simulink model "dspdtmf_audio"  (Simulink 8.3)
settings: Solver=FixedStepDiscrete  SolverMode=SingleTasking  StartTime=0  StopTime=5  RelTol=1e-3
model workspace (MAT data in the model file):
  dtmfFramesize = 256
  dtmfFs : num (value not decoded)
undefined symbols (not defined in the file or in its folder): dfilt, jet
libraries: dspsrcs4 x7, dspsigops x2, dspsnks4 x2, dspobslib x1, dsparch4 x1, dspswit3 x1, dspbuff3 x1, dspmisc x1, dspspect3 x1, dspmathops x1
settings Model: FPTRunName=Active  Creator=The MathWorks Inc.  ExtModeTrigMode=oneshot  ExtModeArmWhenConnect=off  ExtModeAutoUpdateStatusClock=off  BufferReuse=off
settings DataIOCC: LimitDataPoints=off  SaveOutput=off  SignalLogging=off  SaveTime=off
settings OptimizationCC: BlockReduction=off  BooleanDataType=off  OptimizeBlockIOStorage=off  BufferReuse=off  GlobalBufferReuse=off  ExpressionFolding=off  ExpressionDepthLimit=2147483647  FoldNonRolledExpr=off  LocalBlockOutputs=off  InitFltsAndDblsToZero=on
settings DebuggingCC: SignalResolutionControl=TryResolveAllWithWarning  SolverPrmCheckMsg=none  MultiTaskDSMMsg=warning  MultiTaskCondExecSysMsg=none  FcnCallInpInsideContextMsg=UseLocalSettings  StrictBusMsg=None
settings HardwareCC: TargetUnknown=on
settings SFSimCC: SimParseCustomCode=off
settings RTWCC: IncludeERTFirstTime=on
settings GRTTargetCC: TargetFcnLib=ansi_tfl_tmw_new.mat

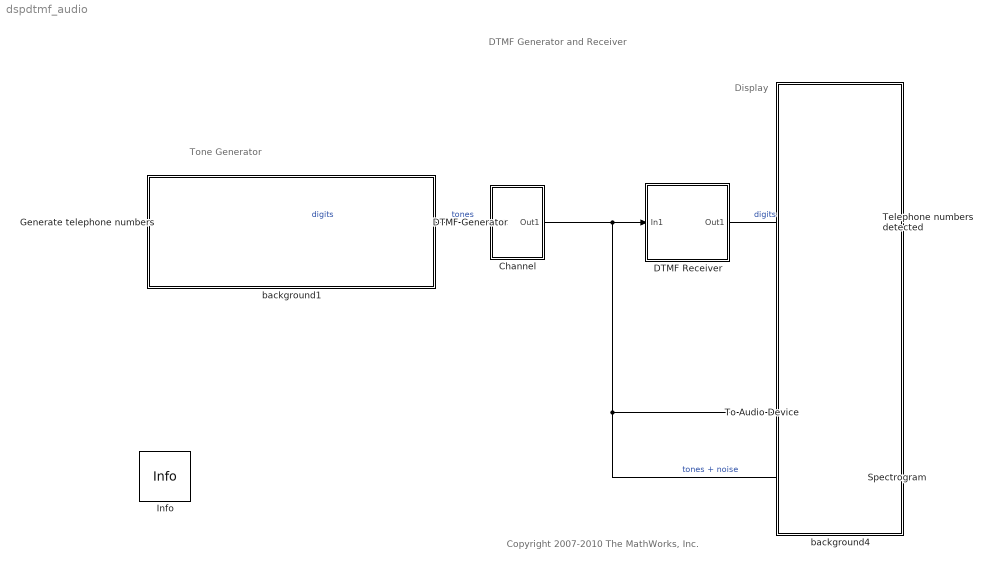
== system dspdtmf_audio ==
  note: DTMF Generator and Receiver
  note: Display
  note: Tone
      | Generator
  note: Copyright 2007-2010 The MathWorks, Inc.
  Channel : Subsystem  mask(Channel){var=0.04, g=2}
      mask prompts: var "Noise power"; g "Gain"
      mask help: Models a noisy channel
      mask Display: disp('Channel')
  DTMF Generator : Subsystem  mask(DTMF Generator){dtmfdelta_f1=4.5, dtmfdelta_f2=0, dtmfdelta_f3=0, dtmfdelta_f4=0, dtmfdelta_f5=0, dtmfdelta_f6=0, dtmfdelta_f7=0}
      mask prompts: dtmfdelta_f1 "Row tone 1 (697 Hz) frequency bias (%):"; dtmfdelta_f2 "Row tone 2 (770 Hz) frequency bias (%):"; dtmfdelta_f3 "Row tone 3 (852 Hz) frequency bias (%):"; dtmfdelta_f4 "Row tone 4 (941 Hz) frequency bias (%):"; dtmfdelta_f5 "Column tone 1 (1209 Hz) frequency bias (%):"; dtmfdelta_f6 "Column tone 2 (1336 Hz) frequency bias (%):"; dtmfdelta_f7 "Column tone 3 (1477 Hz) frequency bias (%):"
      mask help: Generates dual-tone multifrequency tones by summing row and column frequency tones. The frequency bias of each row and column frequency tone can be specified as a percentage of the tone frequency.
      mask Display: disp('DTMF\nGenerator');
  DTMF Receiver : Subsystem  mask(DTMF Receiver){dtmf_p=4.5}
      mask prompts: dtmf_p "Bandpass filter frequency bandwidth (% of central frequency):"
      mask help: Receiver and decoder for dual-tone multifrequency tones. The bandwidth of the bandpass filters can be specified as a percentage of the center frequency.
      mask Display: disp('DTMF\nReceiver');
  Generate telephone numbers : Subsystem  mask{Number=[1 5 0 8 6 4 7 7 0 0 0], Td=(1/dtmfFs)*256*6}
      mask prompts: Number "Telephone number"; Td "Digit Period (s)"
      mask help: This block simulates the dialed numbers. The output is a sequency of pulses with the dialed number as the pulse amplitude.
      mask init:
      | if (~isreal(Number) || ~isvector(Number) || issparse(Number) || ischar(Number) || isfi(Number))
      |     error(['Input must be an integer vector with values in the range 0 to 11, inclusive']);
      | end
      | for i = 1:length(Number)
      |     if ((Number(i) > 11) || (Number(i)<0)) || ((Number(i)-floor(Number(i)))~=0)
      |         error(['Input values must be integers from 0 to 11, inclusive']);
      |     end
      | end
      mask Display: disp(Number)
  Info : dspmisc/Info  SystemSampleTime=-1
  Spectrogram : Subsystem
  Telephone numbers detected : Display
  To Audio Device : dspsnks4/To Audio Device  deviceName=Default  inheritSampleRate=on  sampleRate=44100  deviceDatatype=Determine from input data type  autoBufferSize=on  bufferSize=4096  queueDuration=0.3  defaultOutputChannelMapping=on  outputChannelMapping=1
  background1 : Subsystem
      mask Display: disp('')
  background4 : Subsystem
      mask Display: disp('')
  wires:
  Generate telephone numbers/1(Out1) -> DTMF Generator/1(In1)  "digits"
  Channel/1(Out1) -> DTMF Receiver/1(In1), Spectrogram/1(In1), To Audio Device/1  "tones + noise"
  DTMF Receiver/1(Out1) -> Telephone numbers detected/1  "digits"
  DTMF Generator/1(Out1) -> Channel/1(In1)  "tones"

== system dspdtmf_audio/Channel ==
  In1 : Inport
  Gain : Gain  Gain=g  SaturateOnIntegerOverflow=on  OutDataTypeStr=Inherit: Same as input  ParamDataTypeStr=Inherit: Same as input
  Sum : Sum  Inputs=|++  SaturateOnIntegerOverflow=on  InputSameDT=on  OutDataTypeStr=Inherit: Same as first input
  Vector of Noise : RandomNumber  Variance=var  Seed=[1:dtmfFramesize]  SampleTime=dtmfFramesize/dtmfFs
  Out1 : Outport
  wires:
  In1/1 -> Gain/1
  Gain/1 -> Sum/1
  Vector of Noise/1 -> Sum/2
  Sum/1 -> Out1/1

== system dspdtmf_audio/DTMF Generator ==
  In1 : Inport
  Constant : Constant
  Digit to Tone : Subsystem  TreatAsAtomicUnit=on
  Sum : Sum  Inputs=|+-  SaturateOnIntegerOverflow=on  InputSameDT=on  OutDataTypeStr=Inherit: Same as first input
  Out1 : Outport
  wires:
  In1/1 -> Digit to Tone/Enable, Sum/1
  Sum/1 -> Digit to Tone/1(In1)
  Constant/1 -> Sum/2
  Digit to Tone/1(Out1) -> Out1/1

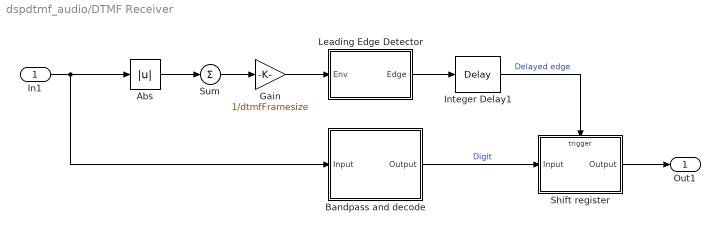
== system dspdtmf_audio/DTMF Receiver ==
  In1 : Inport
  Abs : Abs  SaturateOnIntegerOverflow=on
  Bandpass and decode : Subsystem
  Gain : Gain  Gain=1/dtmfFramesize  SaturateOnIntegerOverflow=on  OutDataTypeStr=Inherit: Same as input  ParamDataTypeStr=Inherit: Same as input
  Integer Delay1 : dspsigops/Delay  dly_unit=Samples  delay=1  ic_detail=off  dif_ic_for_ch=off  dif_ic_for_dly=off  ic=0  reset_popup=None
  Leading Edge Detector : Subsystem
  Shift register : Subsystem  TreatAsAtomicUnit=on
  Sum : Sum  Inputs=1  SaturateOnIntegerOverflow=on  InputSameDT=on  OutDataTypeStr=Inherit: Same as first input
  Out1 : Outport
  wires:
  In1/1 -> Bandpass and decode/1(Input), Abs/1
  Abs/1 -> Sum/1
  Sum/1 -> Gain/1
  Gain/1 -> Leading Edge Detector/1(Env)
  Leading Edge Detector/1(Edge) -> Integer Delay1/1
  Bandpass and decode/1(Output) -> Shift register/1(Input)  "Digit"
  Integer Delay1/1 -> Shift register/Trigger  "Delayed edge"
  Shift register/1(Output) -> Out1/1

== system dspdtmf_audio/Generate telephone numbers ==
  Discrete Pulse Generator : DiscretePulseGenerator  SampleTime=Td
  Product : Product  SaturateOnIntegerOverflow=on  RndMeth=Zero  InputSameDT=on  OutDataTypeStr=Inherit: Same as first input
  Triggered Signal From Workspace1 : dspsigops/Triggered Signal From Workspace  Signal=Number+1  TriggerType=Rising edge  ic=0  SamplesPerFrame=1  OutputAfterFinalValue=Setting to zero
  Out1 : Outport
  wires:
  Discrete Pulse Generator/1 -> Product/1, Triggered Signal From Workspace1/Trigger
  Triggered Signal From Workspace1/1 -> Product/2
  Product/1 -> Out1/1

== system dspdtmf_audio/Spectrogram ==
  In1 : Inport
  Buffer2 : Buffer  N=48*64  V=46*64  ic=-70  TreatMby1Signals=One channel
  Reshape : Reshape  OutputDimensionality=Customize  OutputDimensions=[64 48]
  Selector : Selector  InputPortWidth=dtmfFramesize/2  Indices=1:(dtmfFramesize/4)
  Short-Time FFT1 : dspspect3/Periodogram  measurement=Power spectral density  wintype=Hamming  Rs=50  beta=5  winsamp=Periodic  FFTImplementation=Auto  inheritFFT=off  fftsize=128  navg=2  inheritTs=on  Ts=1
  Spectogram : dspsnks4/Matrix Viewer  ImageParams=on  CMapStr=jet(256)  AxisColorbar=off  AxisParams=on  AxisOrigin=Lower left corner  XLabel=Time Index  YLabel=Frequency Index  ZLabel=dB Magnitude  FigPos=[214 452 283 114]  AxisZoom=on
      settings: YMin=-150  YMax=-65
  dB Conversion : dspmathops/dB Conversion  dBtype=dB  intype=Amplitude  R=1  fuzz=on
  wires:
  Short-Time FFT1/1 -> Selector/1
  Selector/1 -> dB Conversion/1
  Buffer2/1 -> Reshape/1
  In1/1 -> Short-Time FFT1/1
  Reshape/1 -> Spectogram/1
  dB Conversion/1 -> Buffer2/1

== system dspdtmf_audio/background1 ==

== system dspdtmf_audio/background4 ==

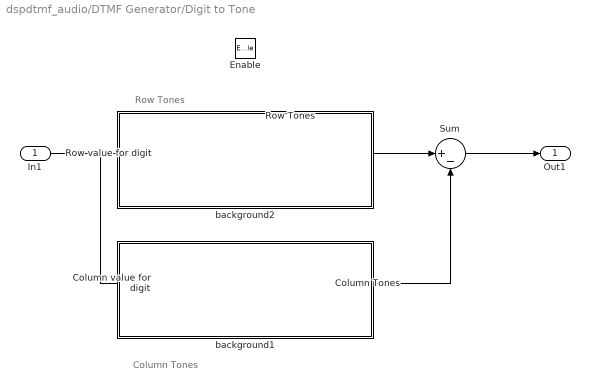
== system dspdtmf_audio/DTMF Generator/Digit to Tone ==
  note: Row Tones
  note: Column Tones
  In1 : Inport
  Enable : EnablePort  PropagateVarSize=During execution
  Column Tones : Subsystem
  Column value for digit : Lookup_n-D  NumberOfTableDimensions=1  BreakpointsForDimension1=[0 1 2 3 4 5 6 7 8 9 10 11]  Table=[1 0 1 2 0 1 2 0 1 2 0 2]  SaturateOnIntegerOverflow=on  InputSameDT=on
  Row Tones : Subsystem
  Row value for digit : Lookup_n-D  NumberOfTableDimensions=1  BreakpointsForDimension1=[0 1 2 3 4 5 6 7 8 9 10 11]  Table=[3 0 0 0 1 1 1 2 2 2 3 3]  SaturateOnIntegerOverflow=on  InputSameDT=on
  Sum : Sum  Inputs=|+-  SaturateOnIntegerOverflow=on  InputSameDT=on  OutDataTypeStr=Inherit: Same as first input
  background1 : Subsystem
      mask Display: disp('')
  background2 : Subsystem
      mask Display: disp('')
  Out1 : Outport  OutputWhenDisabled=reset  InitialOutput=0
  wires:
  Sum/1 -> Out1/1
  Column value for digit/1 -> Column Tones/1(Column)
  Row value for digit/1 -> Row Tones/1(Row)
  In1/1 -> Column value for digit/1, Row value for digit/1
  Column Tones/1(Tone) -> Sum/2
  Row Tones/1(Tone) -> Sum/1

== system dspdtmf_audio/DTMF Receiver/Bandpass and decode ==
  Input : Inport
  Calculate Digit : Lookup_n-D  BreakpointsForDimension1=[1:4]  BreakpointsForDimension2=[1:3]  Table=[1 2 3;4 5 6;7 8 9;10 0 11]  ExtrapMethod=Clip  SaturateOnIntegerOverflow=on  InputSameDT=on
  Calculate Column : Subsystem
  Calculate Row : Subsystem
  Output : Outport
  wires:
  Input/1 -> Calculate Column/1(In1), Calculate Row/1(In1)  "Input Tones"
  Calculate Digit/1 -> Output/1
  Calculate Row/1(Out1) -> Calculate Digit/1
  Calculate Column/1(Out1) -> Calculate Digit/2

== system dspdtmf_audio/DTMF Receiver/Leading Edge Detector ==
  Env : Inport
  Binary To Bipolar : Fcn  Expr=2*u-1
  Constant : Constant  Value=0.5
  Digital Filter : dsparch4/Digital Filter  TypePopup=FIR (all zeros)  IIRFiltStruct=Direct form II transposed  AllPoleFiltStruct=Direct form  FIRFiltStruct=Direct form  CoeffSource=Specify via dialog  NumCoeffs=[ones(1,4) -ones(1,4)]  DenCoeffs=[1 0.1]  BiQuadCoeffs=[1 0.3 0.4 1 0.1 0.2]  LatticeCoeffs=[0.2 0.4]  denIgnore=on  FiltPerSampPopup=One filter per frame  IC=0  ICnum=0  ICden=0  roundingMode=Floor  overflowMode=off  ScaleValues=1  scaleValueFracLength=14  stageInFracLength=15  stageOutFracLength=15  FilterSource=Specify via dialog  dfiltObjectName=dfilt.dffir([1 2 1])
  Edge Detector1 : dspswit3/Edge Detector
  Relational Operator : RelationalOperator  InputSameDT=on
  Rising Edge Start : Fcn  Expr=u>5
  Edge : Outport
  wires:
  Edge Detector1/1 -> Edge/1
  Digital Filter/1 -> Rising Edge Start/1
  Binary To Bipolar/1 -> Digital Filter/1
  Rising Edge Start/1 -> Edge Detector1/1
  Env/1 -> Relational Operator/1
  Constant/1 -> Relational Operator/2
  Relational Operator/1 -> Binary To Bipolar/1

== system dspdtmf_audio/DTMF Receiver/Shift register ==
  Input : Inport
  Trigger : TriggerPort  ZeroCross=off
  Delay Line : dspbuff3/Delay Line  siz=11  ic=0  directfeed=on  enable_output=off  hold_output=off  TreatMby1Signals=One channel
  Output : Outport
  wires:
  Input/1 -> Delay Line/1
  Delay Line/1 -> Output/1

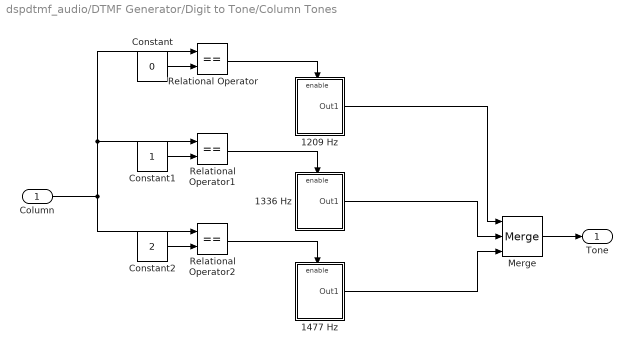
== system dspdtmf_audio/DTMF Generator/Digit to Tone/Column Tones ==
  Column : Inport
  1209 Hz : Subsystem  TreatAsAtomicUnit=on
  1336 Hz : Subsystem  TreatAsAtomicUnit=on
  1477 Hz : Subsystem  TreatAsAtomicUnit=on
  Constant : Constant  Value=0
  Constant1 : Constant
  Constant2 : Constant  Value=2
  Merge : Merge  Inputs=3
  Relational Operator : RelationalOperator  Operator===  InputSameDT=on
  Relational Operator1 : RelationalOperator  Operator===  InputSameDT=on
  Relational Operator2 : RelationalOperator  Operator===  InputSameDT=on
  Tone : Outport
  wires:
  Merge/1 -> Tone/1
  1477 Hz/1(Out1) -> Merge/3
  1336 Hz/1(Out1) -> Merge/2
  1209 Hz/1(Out1) -> Merge/1
  Column/1 -> Relational Operator/1, Relational Operator1/1, Relational Operator2/1
  Relational Operator/1 -> 1209 Hz/Enable
  Relational Operator1/1 -> 1336 Hz/Enable
  Relational Operator2/1 -> 1477 Hz/Enable
  Constant/1 -> Relational Operator/2
  Constant1/1 -> Relational Operator1/2
  Constant2/1 -> Relational Operator2/2

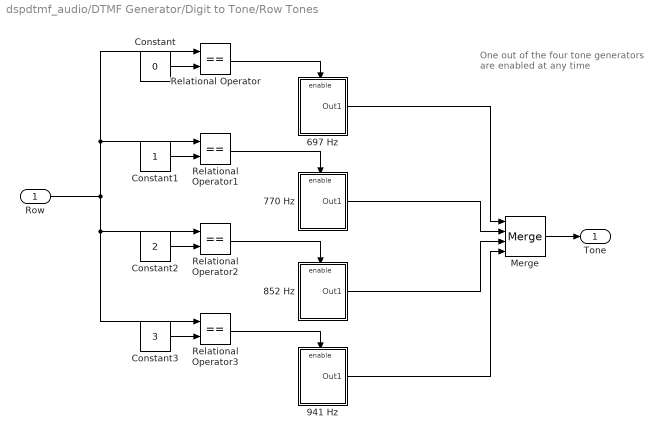
== system dspdtmf_audio/DTMF Generator/Digit to Tone/Row Tones ==
  note: One out of the four tone generators
      | are enabled at any time
  Row : Inport
  697 Hz : Subsystem  TreatAsAtomicUnit=on
  770 Hz : Subsystem  TreatAsAtomicUnit=on
  852 Hz : Subsystem  TreatAsAtomicUnit=on
  941 Hz : Subsystem  TreatAsAtomicUnit=on
  Constant : Constant  Value=0
  Constant1 : Constant
  Constant2 : Constant  Value=2
  Constant3 : Constant  Value=3
  Merge : Merge  Inputs=4
  Relational Operator{,1..3} (4 alike) : RelationalOperator  Operator===  InputSameDT=on
  Tone : Outport
  wires:
  Row/1 -> Relational Operator/1, Relational Operator1/1, Relational Operator2/1, Relational Operator3/1
  697 Hz/1(Out1) -> Merge/1
  770 Hz/1(Out1) -> Merge/2
  852 Hz/1(Out1) -> Merge/3
  941 Hz/1(Out1) -> Merge/4
  Merge/1 -> Tone/1
  Relational Operator/1 -> 697 Hz/Enable
  Relational Operator1/1 -> 770 Hz/Enable
  Relational Operator2/1 -> 852 Hz/Enable
  Relational Operator3/1 -> 941 Hz/Enable
  Constant/1 -> Relational Operator/2
  Constant1/1 -> Relational Operator1/2
  Constant2/1 -> Relational Operator2/2
  Constant3/1 -> Relational Operator3/2

== system dspdtmf_audio/DTMF Generator/Digit to Tone/background1 ==

== system dspdtmf_audio/DTMF Generator/Digit to Tone/background2 ==

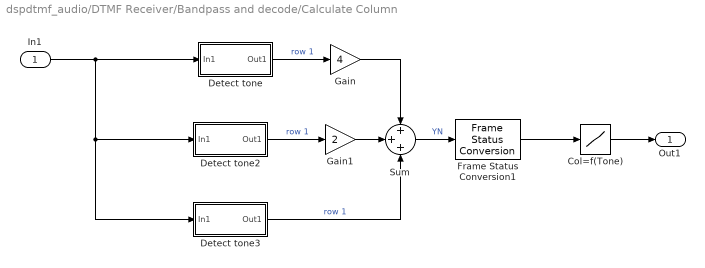
== system dspdtmf_audio/DTMF Receiver/Bandpass and decode/Calculate Column ==
  In1 : Inport
  Col=f(Tone) : Lookup_n-D  NumberOfTableDimensions=1  BreakpointsForDimension1=[0:7]  Table=[0 1 2 0 3 0 0 0]  SaturateOnIntegerOverflow=on  InputSameDT=on
  Detect tone : Subsystem  mask{F=1477}
      mask prompts: F "Frequency"
      settings: AttributesFormatString=%<F> Hz
  Detect tone2 : Subsystem  mask{F=1336}
      mask prompts: F "Frequency"
      settings: AttributesFormatString=%<F> Hz
  Detect tone3 : Subsystem  mask{F=1209}
      mask prompts: F "Frequency"
      settings: AttributesFormatString=%<F> Hz
  Frame Status Conversion1 : dspobslib/Frame Status Conversion  growRefPort=off  outframe=Sample-based
  Gain : Gain  Gain=4
  Gain1 : Gain  Gain=2
  Sum : Sum  Inputs=+++
  Out1 : Outport
  wires:
  Sum/1 -> Frame Status Conversion1/1  "YN"
  Frame Status Conversion1/1 -> Col=f(Tone)/1
  Detect tone2/1(Out1) -> Gain1/1  "row 1"
  In1/1 -> Detect tone/1(In1), Detect tone3/1(In1), Detect tone2/1(In1)
  Col=f(Tone)/1 -> Out1/1
  Gain1/1 -> Sum/2
  Detect tone/1(Out1) -> Gain/1  "row 1"
  Gain/1 -> Sum/1
  Detect tone3/1(Out1) -> Sum/3  "row 1"

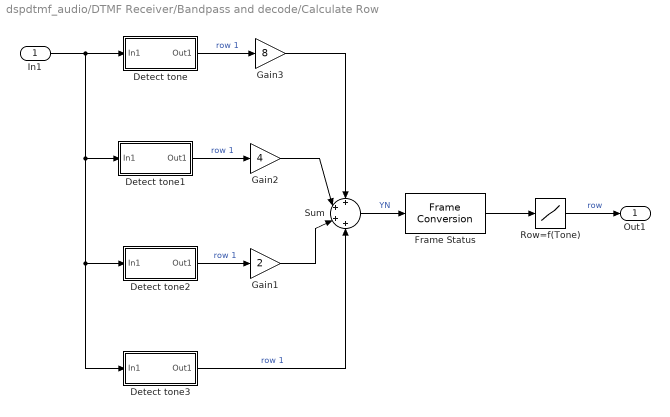
== system dspdtmf_audio/DTMF Receiver/Bandpass and decode/Calculate Row ==
  In1 : Inport
  Detect tone : Subsystem  mask{F=941}
      mask prompts: F "Frequency"
      settings: AttributesFormatString=%<F> Hz
  Detect tone1 : Subsystem  mask{F=852}
      mask prompts: F "Frequency"
      settings: AttributesFormatString=%<F> Hz
  Detect tone2 : Subsystem  mask{F=770}
      mask prompts: F "Frequency"
      settings: AttributesFormatString=%<F> Hz
  Detect tone3 : Subsystem  mask{F=697}
      mask prompts: F "Frequency"
      settings: AttributesFormatString=%<F> Hz
  Frame Status : FrameConversion  OutFrame=Sample-based
  Gain1 : Gain  Gain=2
  Gain2 : Gain  Gain=4
  Gain3 : Gain  Gain=8
  Row=f(Tone) : Lookup_n-D  NumberOfTableDimensions=1  BreakpointsForDimension1=[0:15]  Table=[0 1 2 0 3 0 0 0 4 0 0 0 0 0 0 0]  SaturateOnIntegerOverflow=on  InputSameDT=on
  Sum : Sum  Inputs=++++
  Out1 : Outport
  wires:
  In1/1 -> Detect tone/1(In1), Detect tone1/1(In1), Detect tone2/1(In1), Detect tone3/1(In1)
  Row=f(Tone)/1 -> Out1/1  "row"
  Frame Status/1 -> Row=f(Tone)/1
  Detect tone2/1(Out1) -> Gain1/1  "row 1"
  Detect tone1/1(Out1) -> Gain2/1  "row 1"
  Detect tone/1(Out1) -> Gain3/1  "row 1"
  Gain3/1 -> Sum/1
  Gain2/1 -> Sum/2
  Gain1/1 -> Sum/3
  Sum/1 -> Frame Status/1  "YN"
  Detect tone3/1(Out1) -> Sum/4  "row 1"

== system dspdtmf_audio/DTMF Generator/Digit to Tone/Column Tones/1209 Hz ==
  Enable : EnablePort  PropagateVarSize=During execution
  Sine Wave1 : dspsrcs4/Sine Wave  Amplitude=1  Frequency=1209*(1+dtmfdelta_f5/100)  Phase=0  SampleMode=Discrete  OutComplex=Real  CompMethod=Trigonometric fcn  TableSize=Speed  SampleTime=1/dtmfFs  SamplesPerFrame=dtmfFramesize  ResetState=Restart at time zero  dataType=double  wordLen=16  udDataType=sfix(16)  fracBitsMode=Best precision  numFracBits=15  OutDataTypeStr=double  LastOutDataTypeStr=double
  Out1 : Outport
  wires:
  Sine Wave1/1 -> Out1/1

== system dspdtmf_audio/DTMF Generator/Digit to Tone/Column Tones/1336 Hz ==
  Enable : EnablePort  PropagateVarSize=During execution
  Sine Wave1 : dspsrcs4/Sine Wave  Amplitude=1  Frequency=1336*(1+dtmfdelta_f6/100)  Phase=0  SampleMode=Discrete  OutComplex=Real  CompMethod=Trigonometric fcn  TableSize=Speed  SampleTime=1/dtmfFs  SamplesPerFrame=dtmfFramesize  ResetState=Restart at time zero  dataType=double  wordLen=16  udDataType=sfix(16)  fracBitsMode=Best precision  numFracBits=15  OutDataTypeStr=double  LastOutDataTypeStr=double
  Out1 : Outport
  wires:
  Sine Wave1/1 -> Out1/1

== system dspdtmf_audio/DTMF Generator/Digit to Tone/Column Tones/1477 Hz ==
  Enable : EnablePort  PropagateVarSize=During execution
  Sine Wave1 : dspsrcs4/Sine Wave  Amplitude=1  Frequency=1477*(1+dtmfdelta_f7/100)  Phase=0  SampleMode=Discrete  OutComplex=Real  CompMethod=Trigonometric fcn  TableSize=Speed  SampleTime=1/dtmfFs  SamplesPerFrame=dtmfFramesize  ResetState=Restart at time zero  dataType=double  wordLen=16  udDataType=sfix(16)  fracBitsMode=Best precision  numFracBits=15  OutDataTypeStr=double  LastOutDataTypeStr=double
  Out1 : Outport
  wires:
  Sine Wave1/1 -> Out1/1

== system dspdtmf_audio/DTMF Generator/Digit to Tone/Row Tones/697 Hz ==
  Enable : EnablePort  PropagateVarSize=During execution
  Sine Wave : dspsrcs4/Sine Wave  Amplitude=1  Frequency=697*(1+dtmfdelta_f1/100)  Phase=0  SampleMode=Discrete  OutComplex=Real  CompMethod=Trigonometric fcn  TableSize=Speed  SampleTime=1/dtmfFs  SamplesPerFrame=dtmfFramesize  ResetState=Restart at time zero  dataType=double  wordLen=16  udDataType=sfix(16)  fracBitsMode=Best precision  numFracBits=15  OutDataTypeStr=double  LastOutDataTypeStr=double
  Out1 : Outport
  wires:
  Sine Wave/1 -> Out1/1

== system dspdtmf_audio/DTMF Generator/Digit to Tone/Row Tones/770 Hz ==
  Enable : EnablePort  PropagateVarSize=During execution
  Sine Wave : dspsrcs4/Sine Wave  Amplitude=1  Frequency=770*(1+dtmfdelta_f2/100)  Phase=0  SampleMode=Discrete  OutComplex=Real  CompMethod=Trigonometric fcn  TableSize=Speed  SampleTime=1/dtmfFs  SamplesPerFrame=dtmfFramesize  ResetState=Restart at time zero  dataType=double  wordLen=16  udDataType=sfix(16)  fracBitsMode=Best precision  numFracBits=15  OutDataTypeStr=double  LastOutDataTypeStr=double
  Out1 : Outport
  wires:
  Sine Wave/1 -> Out1/1

== system dspdtmf_audio/DTMF Generator/Digit to Tone/Row Tones/852 Hz ==
  Enable : EnablePort  PropagateVarSize=During execution
  Sine Wave : dspsrcs4/Sine Wave  Amplitude=1  Frequency=852*(1+dtmfdelta_f3/100)  Phase=0  SampleMode=Discrete  OutComplex=Real  CompMethod=Trigonometric fcn  TableSize=Speed  SampleTime=1/dtmfFs  SamplesPerFrame=dtmfFramesize  ResetState=Restart at time zero  dataType=double  wordLen=16  udDataType=sfix(16)  fracBitsMode=Best precision  numFracBits=15  OutDataTypeStr=double  LastOutDataTypeStr=double
  Out1 : Outport
  wires:
  Sine Wave/1 -> Out1/1

== system dspdtmf_audio/DTMF Generator/Digit to Tone/Row Tones/941 Hz ==
  Enable : EnablePort  PropagateVarSize=During execution
  Sine Wave : dspsrcs4/Sine Wave  Amplitude=1  Frequency=941*(1+dtmfdelta_f4/100)  Phase=0  SampleMode=Discrete  OutComplex=Real  CompMethod=Trigonometric fcn  TableSize=Speed  SampleTime=1/dtmfFs  SamplesPerFrame=dtmfFramesize  ResetState=Restart at time zero  dataType=double  wordLen=16  udDataType=sfix(16)  fracBitsMode=Best precision  numFracBits=15  OutDataTypeStr=double  LastOutDataTypeStr=double
  Out1 : Outport
  wires:
  Sine Wave/1 -> Out1/1

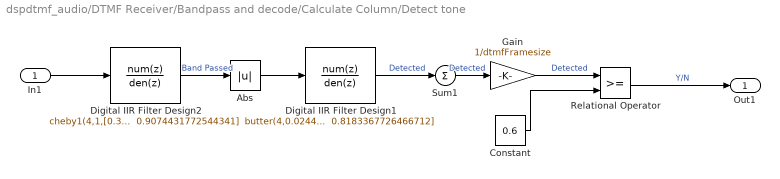
== system dspdtmf_audio/DTMF Receiver/Bandpass and decode/Calculate Column/Detect tone ==
  In1 : Inport
  Abs : Abs  SaturateOnIntegerOverflow=on
  Constant : Constant  Value=0.6
  Digital IIR Filter Design1 : DiscreteFilter  Numerator=butter(4,0.024414 )  Denominator="[1     -3.799600047139706      5.418636382695164      -3.43734174118743     0.8183367726466712]"  InputProcessing=Columns as channels (frame based)
  Digital IIR Filter Design2 : DiscreteFilter  Numerator=cheby1(4,1,[0.34437 0.37682] )  Denominator="[1     -3.351534504625169       8.10699128745984     -12.15068111449483      14.40624674632962     -11.85923479241394      7.722756593485457     -3.116033501354059     0.9074431772544341]"  InputProcessing=Columns as channels (frame based)
  Gain : Gain  Gain=1/dtmfFramesize  SaturateOnIntegerOverflow=on  OutDataTypeStr=Inherit: Same as input  ParamDataTypeStr=Inherit: Same as input
  Relational Operator : RelationalOperator  InputSameDT=on
  Sum1 : Sum  Inputs=1  SaturateOnIntegerOverflow=on  InputSameDT=on  OutDataTypeStr=Inherit: Same as first input
  Out1 : Outport
  wires:
  Digital IIR Filter Design1/1 -> Sum1/1  "Detected"
  Relational Operator/1 -> Out1/1  "Y/N"
  Constant/1 -> Relational Operator/2
  Abs/1 -> Digital IIR Filter Design1/1
  Digital IIR Filter Design2/1 -> Abs/1  "Band Passed"
  In1/1 -> Digital IIR Filter Design2/1
  Sum1/1 -> Gain/1  "Detected"
  Gain/1 -> Relational Operator/1  "Detected"

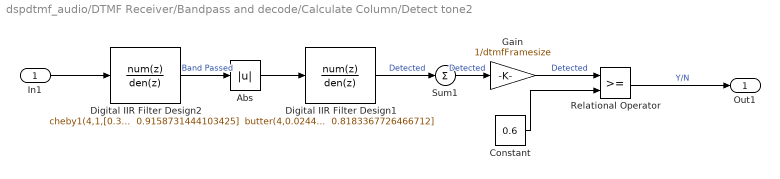
== system dspdtmf_audio/DTMF Receiver/Bandpass and decode/Calculate Column/Detect tone2 ==
  In1 : Inport
  Abs : Abs  SaturateOnIntegerOverflow=on
  Constant : Constant  Value=0.6
  Digital IIR Filter Design1 : DiscreteFilter  Numerator=butter(4,0.024414 )  Denominator="[1     -3.799600047139706      5.418636382695164      -3.43734174118743     0.8183367726466712]"  InputProcessing=Columns as channels (frame based)
  Digital IIR Filter Design2 : DiscreteFilter  Numerator=cheby1(4,1,[0.31149 0.34085] )  Denominator="[1     -4.109271737397858      10.23854068371831     -16.38274148509198      19.22475767149518     -16.02675157800493      9.798412568107882     -3.847129397590863     0.9158731444103425]"  InputProcessing=Columns as channels (frame based)
  Gain : Gain  Gain=1/dtmfFramesize  SaturateOnIntegerOverflow=on  OutDataTypeStr=Inherit: Same as input  ParamDataTypeStr=Inherit: Same as input
  Relational Operator : RelationalOperator  InputSameDT=on
  Sum1 : Sum  Inputs=1  SaturateOnIntegerOverflow=on  InputSameDT=on  OutDataTypeStr=Inherit: Same as first input
  Out1 : Outport
  wires:
  Gain/1 -> Relational Operator/1  "Detected"
  Sum1/1 -> Gain/1  "Detected"
  In1/1 -> Digital IIR Filter Design2/1
  Digital IIR Filter Design2/1 -> Abs/1  "Band Passed"
  Abs/1 -> Digital IIR Filter Design1/1
  Constant/1 -> Relational Operator/2
  Relational Operator/1 -> Out1/1  "Y/N"
  Digital IIR Filter Design1/1 -> Sum1/1  "Detected"

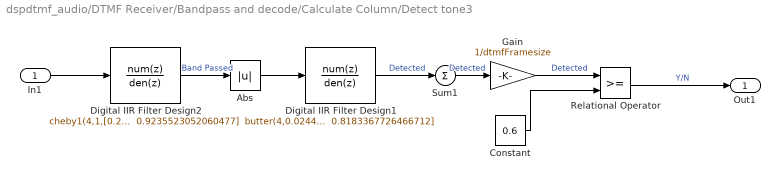
== system dspdtmf_audio/DTMF Receiver/Bandpass and decode/Calculate Column/Detect tone3 ==
  In1 : Inport
  Abs : Abs  SaturateOnIntegerOverflow=on
  Constant : Constant  Value=0.6
  Digital IIR Filter Design1 : DiscreteFilter  Numerator=butter(4,0.024414 )  Denominator="[1     -3.799600047139706      5.418636382695164      -3.43734174118743     0.8183367726466712]"  InputProcessing=Columns as channels (frame based)
  Digital IIR Filter Design2 : DiscreteFilter  Numerator=cheby1(4,1,[0.28188 0.30845] )  Denominator="[1     -4.752348043106542      12.38564406749955     -20.67287188883259      24.34715829142214     -20.26589425714094      11.90277663892072     -4.477143154545357     0.9235523052060477]"  InputProcessing=Columns as channels (frame based)
  Gain : Gain  Gain=1/dtmfFramesize  SaturateOnIntegerOverflow=on  OutDataTypeStr=Inherit: Same as input  ParamDataTypeStr=Inherit: Same as input
  Relational Operator : RelationalOperator  InputSameDT=on
  Sum1 : Sum  Inputs=1  SaturateOnIntegerOverflow=on  InputSameDT=on  OutDataTypeStr=Inherit: Same as first input
  Out1 : Outport
  wires:
  Digital IIR Filter Design1/1 -> Sum1/1  "Detected"
  Relational Operator/1 -> Out1/1  "Y/N"
  Constant/1 -> Relational Operator/2
  Abs/1 -> Digital IIR Filter Design1/1
  Digital IIR Filter Design2/1 -> Abs/1  "Band Passed"
  In1/1 -> Digital IIR Filter Design2/1
  Sum1/1 -> Gain/1  "Detected"
  Gain/1 -> Relational Operator/1  "Detected"

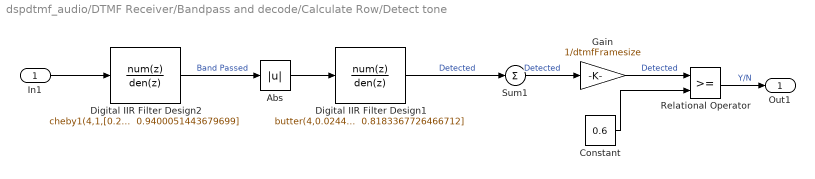
== system dspdtmf_audio/DTMF Receiver/Bandpass and decode/Calculate Row/Detect tone ==
  In1 : Inport
  Abs : Abs  SaturateOnIntegerOverflow=on
  Constant : Constant  Value=0.6
  Digital IIR Filter Design1 : DiscreteFilter  Numerator=butter(4,0.024414 )  Denominator="[1     -3.799600047139706      5.418636382695164      -3.43734174118743     0.8183367726466712]"  InputProcessing=Columns as channels (frame based)
  Digital IIR Filter Design2 : DiscreteFilter  Numerator=cheby1(4,1,[0.2194 0.24007] )  Denominator="[1     -5.958859496378779      17.25206476391561     -30.82030278001819      36.95597582617549     -30.34721652315746      16.72649806780964     -5.688650155299636     0.9400051443679699]"  InputProcessing=Columns as channels (frame based)
  Gain : Gain  Gain=1/dtmfFramesize  SaturateOnIntegerOverflow=on  OutDataTypeStr=Inherit: Same as input  ParamDataTypeStr=Inherit: Same as input
  Relational Operator : RelationalOperator  InputSameDT=on
  Sum1 : Sum  Inputs=1  SaturateOnIntegerOverflow=on  InputSameDT=on  OutDataTypeStr=Inherit: Same as first input
  Out1 : Outport
  wires:
  Gain/1 -> Relational Operator/1  "Detected"
  Sum1/1 -> Gain/1  "Detected"
  In1/1 -> Digital IIR Filter Design2/1
  Digital IIR Filter Design2/1 -> Abs/1  "Band Passed"
  Abs/1 -> Digital IIR Filter Design1/1
  Constant/1 -> Relational Operator/2
  Relational Operator/1 -> Out1/1  "Y/N"
  Digital IIR Filter Design1/1 -> Sum1/1  "Detected"

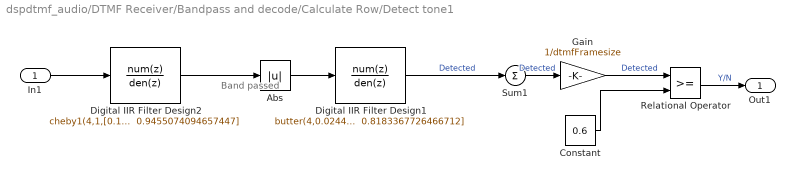
== system dspdtmf_audio/DTMF Receiver/Bandpass and decode/Calculate Row/Detect tone1 ==
  note: Band passed
  In1 : Inport
  Abs : Abs  SaturateOnIntegerOverflow=on
  Constant : Constant  Value=0.6
  Digital IIR Filter Design1 : DiscreteFilter  Numerator=butter(4,0.024414 )  Denominator="[1     -3.799600047139706      5.418636382695164      -3.43734174118743     0.8183367726466712]"  InputProcessing=Columns as channels (frame based)
  Digital IIR Filter Design2 : DiscreteFilter  Numerator=cheby1(4,1,[0.19865 0.21737] )  Denominator="[1     -6.307290738785874      18.86115258817615     -34.33641523909546      41.43128366098485     -33.85873013586509       18.3400163783615     -6.047701819053891     0.9455074094657447]"  InputProcessing=Columns as channels (frame based)
  Gain : Gain  Gain=1/dtmfFramesize  SaturateOnIntegerOverflow=on  OutDataTypeStr=Inherit: Same as input  ParamDataTypeStr=Inherit: Same as input
  Relational Operator : RelationalOperator  InputSameDT=on
  Sum1 : Sum  Inputs=1  SaturateOnIntegerOverflow=on  InputSameDT=on  OutDataTypeStr=Inherit: Same as first input
  Out1 : Outport
  wires:
  Digital IIR Filter Design1/1 -> Sum1/1  "Detected"
  Relational Operator/1 -> Out1/1  "Y/N"
  Constant/1 -> Relational Operator/2
  Abs/1 -> Digital IIR Filter Design1/1
  Digital IIR Filter Design2/1 -> Abs/1
  In1/1 -> Digital IIR Filter Design2/1
  Sum1/1 -> Gain/1  "Detected"
  Gain/1 -> Relational Operator/1  "Detected"

== system dspdtmf_audio/DTMF Receiver/Bandpass and decode/Calculate Row/Detect tone2 ==
  In1 : Inport
  Abs : Abs  SaturateOnIntegerOverflow=on
  Constant : Constant  Value=0.6
  Digital IIR Filter Design1 : DiscreteFilter  Numerator=butter(4,0.024414 )  Denominator="[1     -3.799600047139706      5.418636382695164      -3.43734174118743     0.8183367726466712]"  InputProcessing=Columns as channels (frame based)
  Digital IIR Filter Design2 : DiscreteFilter  Numerator=cheby1(4,1,[0.17953 0.19645] )  Denominator="[1     -6.602847127805465      20.29779156008288     -37.54784384124043      45.55694442771227     -37.07539184815035      19.79020814600772     -6.356732018737127     0.9506151081795299]"  InputProcessing=Columns as channels (frame based)
  Gain : Gain  Gain=1/dtmfFramesize  SaturateOnIntegerOverflow=on  OutDataTypeStr=Inherit: Same as input  ParamDataTypeStr=Inherit: Same as input
  Relational Operator : RelationalOperator  InputSameDT=on
  Sum1 : Sum  Inputs=1  SaturateOnIntegerOverflow=on  InputSameDT=on  OutDataTypeStr=Inherit: Same as first input
  Out1 : Outport
  wires:
  Gain/1 -> Relational Operator/1  "Detected"
  Sum1/1 -> Gain/1  "Detected"
  In1/1 -> Digital IIR Filter Design2/1
  Digital IIR Filter Design2/1 -> Abs/1  "Band Passed"
  Abs/1 -> Digital IIR Filter Design1/1
  Constant/1 -> Relational Operator/2
  Relational Operator/1 -> Out1/1  "Y/N"
  Digital IIR Filter Design1/1 -> Sum1/1  "Detected"

== system dspdtmf_audio/DTMF Receiver/Bandpass and decode/Calculate Row/Detect tone3 ==
  In1 : Inport
  Abs : Abs  SaturateOnIntegerOverflow=on
  Constant : Constant  Value=0.6
  Digital IIR Filter Design1 : DiscreteFilter  Numerator=butter(4,0.024414 )  Denominator="[1     -3.799600047139706      5.418636382695164      -3.43734174118743     0.8183367726466712]"  InputProcessing=Columns as channels (frame based)
  Digital IIR Filter Design2 : DiscreteFilter  Numerator=cheby1(4,1,[0.16251 0.17782] )  Denominator="[1     -6.844396697786066      21.52092460865172     -40.33641962283424      49.16722309158686     -39.87689970998925      21.03338086634554     -6.613139526612567     0.9552071096321408]"  InputProcessing=Columns as channels (frame based)
  Gain : Gain  Gain=1/dtmfFramesize  SaturateOnIntegerOverflow=on  OutDataTypeStr=Inherit: Same as input  ParamDataTypeStr=Inherit: Same as input
  Relational Operator : RelationalOperator  InputSameDT=on
  Sum1 : Sum  Inputs=1  SaturateOnIntegerOverflow=on  InputSameDT=on  OutDataTypeStr=Inherit: Same as first input
  Out1 : Outport
  wires:
  Digital IIR Filter Design1/1 -> Sum1/1  "Detected"
  Relational Operator/1 -> Out1/1  "Y/N"
  Constant/1 -> Relational Operator/2
  Abs/1 -> Digital IIR Filter Design1/1
  Digital IIR Filter Design2/1 -> Abs/1  "Band Passed"
  In1/1 -> Digital IIR Filter Design2/1
  Sum1/1 -> Gain/1  "Detected"
  Gain/1 -> Relational Operator/1  "Detected"
